simulink model "gm_sampleModel1890_2_sub"  (R2023a)
settings: Solver=VariableStepAuto  StartTime=0.0  StopTime=10.0  RelTol=1e-3
settings Model: Creator=user1  LastModifiedBy=user1
settings OptimizationCC: BlockReduction=off  ConditionallyExecuteInputs=off
settings DebuggingCC: InheritedTsInSrcMsg=none

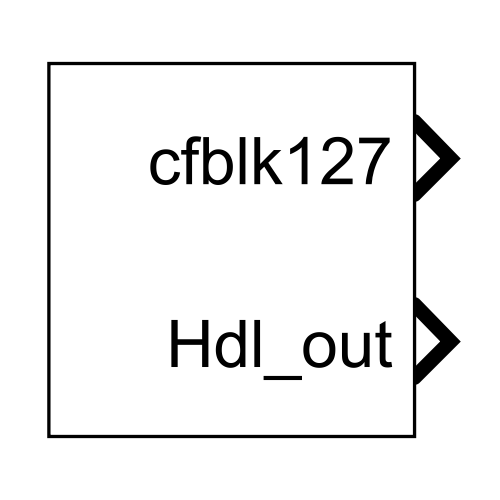
[thumbnail: Simulink's stored preview of the top-level diagram]
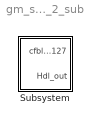
== system gm_sampleModel1890_2_sub ==
  Subsystem : Subsystem

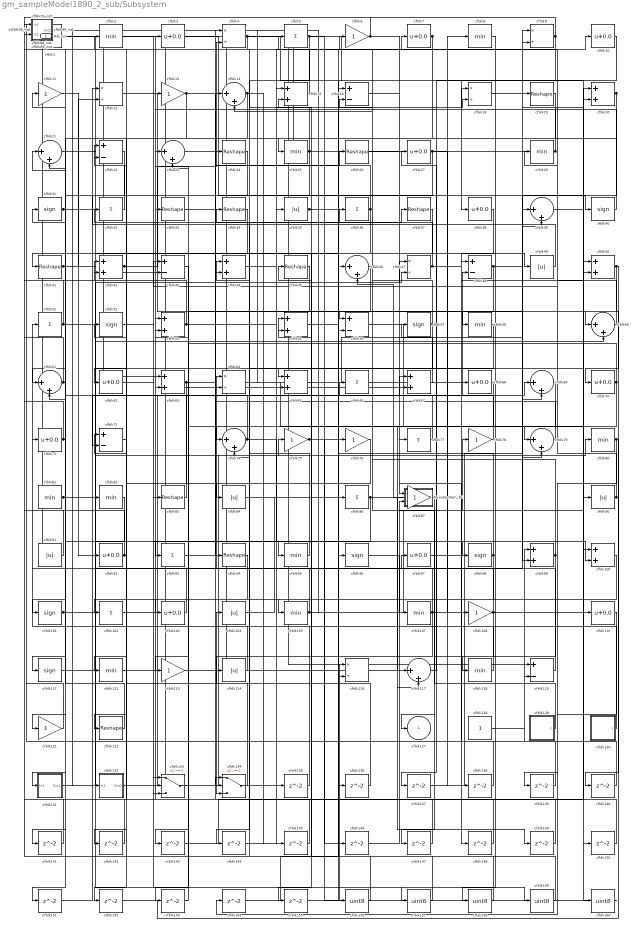
== system gm_sampleModel1890_2_sub/Subsystem ==
  Mysubsystem_36 : Subsystem
  cfblk{1,5,32,36,51,66,77,86,93,102} (10 alike) : Sum  Inputs=+  OutDataTypeStr=uint8
  cfblk{3,7,10,27,38,62,68,70..71,92,97,103,110} (13 alike) : Bias  Bias=0.0  SaturateOnIntegerOverflow=off
  cfblk{15,20,42,44,50,53,55,63,65,67,99..100} (12 alike) : Sum  OutDataTypeStr=uint8
  cfblk{31,40,52,57,96,98,101,111} (8 alike) : Signum
  cfblk{35,49,84,90..91,104,114} (7 alike) : Abs  OutDataTypeStr=uint8  SaturateOnIntegerOverflow=off
  cfblk{2,8,25,29,58,80..82,95,105,107,112,118} (13 alike) : MinMax  OutDataTypeStr=uint8
  cfblk{6,11,13,75..76,78,87,108,113,121} (10 alike) : Gain  OutDataTypeStr=uint8
  cfblk109_inst : Subsystem
  cfblk115_inst : Subsystem
  cfblk{4,9,12,18,47,64,116} (7 alike) : Product  Inputs=*/  OutDataTypeStr=uint8  RndMeth=Zero  SaturateOnIntegerOverflow=on
  cfblk{14,21,23,39,46,60..61,69,74,79,117} (11 alike) : Sum  Inputs=|++  OutDataTypeStr=uint8
  cfblk{16,22,43,48,56,72,119} (7 alike) : Sum  Inputs=+-  OutDataTypeStr=uint8
  cfblk120_inst : Subsystem
  cfblk{19,24,26,33..34,37,41,45,83,94,122} (11 alike) : Reshape
  cfblk128 : Constant  OutDataTypeStr=uint8  SampleTime=-1
  cfblk129 : Subsystem  mask(Counter Free-Running){NumBits=double(16), tsamp=double(-1)}
      mask prompts: NumBits "Simulink:masks:NumberOfBits_MP"; tsamp "Simulink:masks:SampleTime_MP"
      mask help: Simulink:masks:CounterFreeRunning_MD
  cfblk130 : Subsystem  mask(Counter Free-Running){NumBits=double(16), tsamp=double(-1)}
      mask prompts: NumBits "Simulink:masks:NumberOfBits_MP"; tsamp "Simulink:masks:SampleTime_MP"
      mask help: Simulink:masks:CounterFreeRunning_MD
  cfblk131 : Subsystem
  cfblk132 : Subsystem
  cfblk133 : Switch  OutDataTypeStr=uint8  SaturateOnIntegerOverflow=off  InputSameDT=off
  cfblk134 : Switch  OutDataTypeStr=uint8  SaturateOnIntegerOverflow=off  InputSameDT=off
  cfblk{135..155} (21 alike) : Delay  SampleTime=1
  cfblk{156..160} (5 alike) : DataTypeConversion  OutDataTypeStr=uint8  SaturateOnIntegerOverflow=off  RndMeth=Floor
  cfblk17_inst : Subsystem
  cfblk30_inst : Subsystem
  cfblk59_inst : Subsystem
  cfblk73_inst : Subsystem
  cfblk85_inst : Subsystem
  cfblk88_inst : Subsystem
  cfblk89_inst : Subsystem
  cfblk127 : Outport  OutDataTypeStr=uint8  SampleTime=1  VectorParamsAs1DForOutWhenUnconnected=off
  Hdl_out : Outport  Port=2  OutDataTypeStr=uint8  SampleTime=1
  wires:
  Mysubsystem_36/1(cfblk127) -> cfblk127/1
  cfblk1/1 -> cfblk159/1
  cfblk10/1 -> cfblk137/1
  cfblk100/1 -> cfblk105/1
  cfblk101/1 -> cfblk60/2, cfblk75/1, cfblk47/2
  cfblk102/1 -> cfblk3/1
  cfblk103/1 -> cfblk53/1
  cfblk104/1 -> cfblk86/1
  cfblk105/1 -> cfblk78/1, cfblk51/1
  cfblk107/1 -> cfblk15/2, cfblk134/3, cfblk8/1
  cfblk108/1 -> cfblk64/1, cfblk147/1
  cfblk109_inst/1(out1) -> cfblk63/1
  cfblk11/1 -> cfblk92/1
  cfblk110/1 -> cfblk154/1
  cfblk111/1 -> Mysubsystem_36/2(In2)
  cfblk112/1 -> cfblk97/1
  cfblk113/1 -> cfblk80/1
  cfblk114/1 -> cfblk71/1
  cfblk115_inst/1(out1) -> cfblk117/1
  cfblk116/1 -> cfblk87/1
  cfblk117/1 -> cfblk27/1
  cfblk118/1 -> cfblk61/2
  cfblk119/1 -> cfblk45/1
  cfblk12/1 -> cfblk56/1
  cfblk120_inst/1(out1) -> cfblk135/1
  cfblk121/1 -> cfblk85_inst/1(in1)
  cfblk122/1 -> cfblk11/1
  cfblk128/1 -> cfblk99/1
  cfblk129/1(y) -> cfblk36/1
  cfblk13/1 -> cfblk94/1, cfblk152/1
  cfblk130/1(y) -> cfblk44/1
  cfblk131/1(Out1) -> cfblk35/1
  cfblk132/1(Out1) -> cfblk48/2
  cfblk133/1 -> cfblk39/1
  cfblk134/1 -> cfblk104/1
  cfblk135/1 -> cfblk42/1
  cfblk136/1 -> cfblk72/1
  cfblk137/1 -> cfblk9/2
  cfblk138/1 -> cfblk115_inst/2(in2)
  cfblk139/1 -> cfblk48/1
  cfblk14/1 -> cfblk21/2, cfblk145/1
  cfblk140/1 -> cfblk119/2
  cfblk141/1 -> cfblk109_inst/1(in1)
  cfblk142/1 -> cfblk59_inst/1(in1)
  cfblk143/1 -> cfblk20/2
  cfblk144/1 -> cfblk18/2
  cfblk145/1 -> cfblk22/1
  cfblk146/1 -> cfblk50/2
  cfblk147/1 -> cfblk63/2
  cfblk148/1 -> cfblk134/1
  cfblk149/1 -> cfblk89_inst/2(in2)
  cfblk15/1 -> cfblk73_inst/1(in1)
  cfblk150/1 -> cfblk23/1
  cfblk151/1 -> cfblk69/1
  cfblk152/1 -> cfblk60/1
  cfblk153/1 -> cfblk53/2
  cfblk154/1 -> cfblk46/1
  cfblk155/1 -> cfblk116/1
  cfblk156/1 -> cfblk34/1
  cfblk157/1 -> cfblk55/1
  cfblk158/1 -> cfblk55/2
  cfblk159/1 -> cfblk109_inst/2(in2)
  cfblk16/1 -> cfblk77/1
  cfblk160/1 -> cfblk1/1
  cfblk17_inst/1(out1) -> cfblk30_inst/2(in2)
  cfblk18/1 -> cfblk19/1
  cfblk19/1 -> cfblk62/1
  cfblk2/1 -> cfblk133/1
  cfblk20/1 -> cfblk99/2, cfblk25/1
  cfblk21/1 -> cfblk136/1
  cfblk22/1 -> cfblk72/2
  cfblk23/1 -> cfblk44/2
  cfblk24/1 -> cfblk131/1(In1)
  cfblk25/1 -> cfblk30_inst/1(in1), cfblk122/1
  cfblk26/1 -> cfblk40/1
  cfblk27/1 -> cfblk84/1, cfblk138/1
  cfblk29/1 -> cfblk13/1, Hdl_out/1
  cfblk3/1 -> cfblk69/2
  cfblk30_inst/1(out1) -> cfblk91/1
  cfblk31/1 -> cfblk76/1, cfblk121/1
  cfblk32/1 -> cfblk22/2
  cfblk33/1 -> cfblk26/1
  cfblk34/1 -> cfblk141/1
  cfblk35/1 -> cfblk79/1, cfblk100/2
  cfblk36/1 -> cfblk41/1, cfblk16/2, cfblk4/2
  cfblk37/1 -> cfblk65/1
  cfblk38/1 -> cfblk61/1
  cfblk39/1 -> cfblk90/1
  cfblk4/1 -> cfblk96/1, cfblk85_inst/2(in2), cfblk150/1
  cfblk40/1 -> cfblk14/1
  cfblk41/1 -> cfblk160/1, cfblk12/2
  cfblk42/1 -> cfblk79/2, cfblk24/1
  cfblk43/1 -> cfblk143/1
  cfblk44/1 -> cfblk7/1
  cfblk45/1 -> cfblk103/1
  cfblk46/1 -> cfblk95/1
  cfblk47/1 -> cfblk49/1, cfblk4/1, cfblk2/1
  cfblk48/1 -> cfblk56/2, cfblk20/1
  cfblk49/1 -> cfblk12/1
  cfblk5/1 -> cfblk38/1, cfblk144/1
  cfblk50/1 -> cfblk70/1, cfblk93/1
  cfblk51/1 -> cfblk73_inst/2(in2), cfblk114/1
  cfblk52/1 -> cfblk157/1
  cfblk53/1 -> cfblk120_inst/1(in1), cfblk18/1
  cfblk55/1 -> cfblk156/1
  cfblk56/1 -> cfblk100/1
  cfblk57/1 -> cfblk74/2, cfblk17_inst/2(in2), cfblk14/2
  cfblk58/1 -> cfblk155/1
  cfblk59_inst/1(out1) -> cfblk110/1, cfblk132/1(In1)
  cfblk6/1 -> cfblk17_inst/1(in1), cfblk148/1
  cfblk60/1 -> cfblk29/1
  cfblk61/1 -> cfblk21/1, cfblk120_inst/2(in2)
  cfblk62/1 -> cfblk83/1
  cfblk63/1 -> cfblk47/1, cfblk102/1
  cfblk64/1 -> cfblk117/2
  cfblk65/1 -> cfblk39/2
  cfblk66/1 -> Mysubsystem_36/1(In1)
  cfblk67/1 -> cfblk57/1
  cfblk68/1 -> cfblk74/1
  cfblk69/1 -> cfblk116/2
  cfblk7/1 -> cfblk134/2, cfblk101/1
  cfblk70/1 -> cfblk23/2, cfblk113/1
  cfblk71/1 -> cfblk88_inst/2(in2), cfblk151/1
  cfblk72/1 -> cfblk42/2
  cfblk73_inst/1(out1) -> cfblk67/2, cfblk65/2
  cfblk74/1 -> cfblk98/1, cfblk33/1
  cfblk75/1 -> cfblk67/1, cfblk146/1
  cfblk76/1 -> cfblk112/1
  cfblk77/1 -> cfblk52/1
  cfblk78/1 -> cfblk15/1
  cfblk79/1 -> cfblk9/1
  cfblk8/1 -> cfblk158/1
  cfblk80/1 -> cfblk140/1, cfblk139/1
  cfblk81/1 -> cfblk108/1, cfblk82/1
  cfblk82/1 -> cfblk111/1
  cfblk83/1 -> cfblk59_inst/2(in2)
  cfblk84/1 -> cfblk10/1
  cfblk85_inst/1(out1) -> cfblk43/2, cfblk81/1
  cfblk86/1 -> cfblk133/2, cfblk6/1, cfblk149/1
  cfblk87/1 -> cfblk46/2
  cfblk88_inst/1(out1) -> cfblk68/1
  cfblk89_inst/1(out1) -> cfblk119/1
  cfblk9/1 -> cfblk89_inst/1(in1), cfblk58/1
  cfblk90/1 -> cfblk43/1, cfblk64/2, cfblk5/1
  cfblk91/1 -> cfblk115_inst/1(in1)
  cfblk92/1 -> cfblk88_inst/1(in1), cfblk31/1
  cfblk93/1 -> cfblk37/1
  cfblk94/1 -> cfblk153/1
  cfblk95/1 -> cfblk32/1
  cfblk96/1 -> cfblk107/1
  cfblk97/1 -> cfblk50/1
  cfblk98/1 -> cfblk16/1, cfblk133/3, cfblk142/1
  cfblk99/1 -> cfblk118/1, cfblk66/1

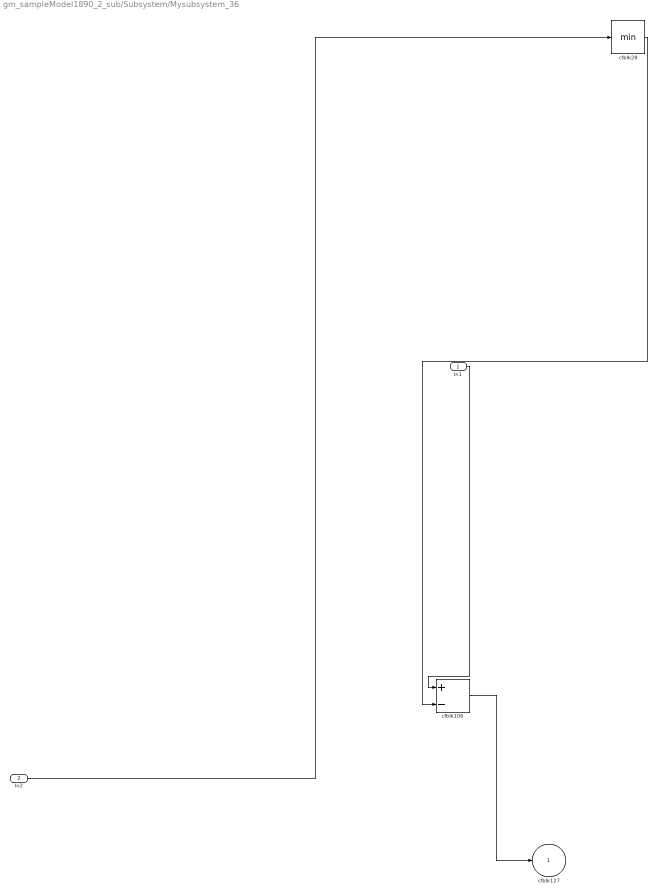
== system gm_sampleModel1890_2_sub/Subsystem/Mysubsystem_36 ==
  In1 : Inport  OutDataTypeStr=uint8  PortDimensions=1  SampleTime=1
  In2 : Inport  Port=2  OutDataTypeStr=uint8  PortDimensions=1  SampleTime=1
  cfblk106 : Sum  Inputs=+-
  cfblk28 : MinMax
  cfblk127 : Outport  SampleTime=1  VectorParamsAs1DForOutWhenUnconnected=off
  wires:
  In1/1 -> cfblk106/1
  In2/1 -> cfblk28/1
  cfblk106/1 -> cfblk127/1
  cfblk28/1 -> cfblk106/2

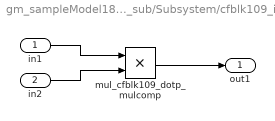
== system gm_sampleModel1890_2_sub/Subsystem/cfblk109_inst ==
  in1 : Inport  OutDataTypeStr=uint8  SampleTime=1
  in2 : Inport  Port=2  OutDataTypeStr=uint8  SampleTime=1
  mul_cfblk109_dotp_mulcomp : Product  Inputs=**  OutDataTypeStr=uint8  SampleTime=1
  out1 : Outport  OutDataTypeStr=uint8  SampleTime=1
  wires:
  in1/1 -> mul_cfblk109_dotp_mulcomp/1
  in2/1 -> mul_cfblk109_dotp_mulcomp/2
  mul_cfblk109_dotp_mulcomp/1 -> out1/1

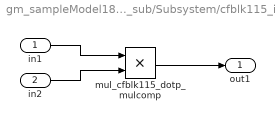
== system gm_sampleModel1890_2_sub/Subsystem/cfblk115_inst ==
  in1 : Inport  OutDataTypeStr=uint8  SampleTime=1
  in2 : Inport  Port=2  OutDataTypeStr=uint8  SampleTime=1
  mul_cfblk115_dotp_mulcomp : Product  Inputs=**  OutDataTypeStr=uint8  SampleTime=1
  out1 : Outport  OutDataTypeStr=uint8  SampleTime=1
  wires:
  in1/1 -> mul_cfblk115_dotp_mulcomp/1
  in2/1 -> mul_cfblk115_dotp_mulcomp/2
  mul_cfblk115_dotp_mulcomp/1 -> out1/1

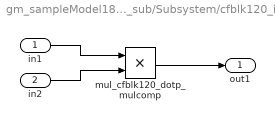
== system gm_sampleModel1890_2_sub/Subsystem/cfblk120_inst ==
  in1 : Inport  OutDataTypeStr=uint8  SampleTime=1
  in2 : Inport  Port=2  OutDataTypeStr=uint8  SampleTime=1
  mul_cfblk120_dotp_mulcomp : Product  Inputs=**  OutDataTypeStr=uint8  SampleTime=1
  out1 : Outport  OutDataTypeStr=uint8  SampleTime=1
  wires:
  in1/1 -> mul_cfblk120_dotp_mulcomp/1
  in2/1 -> mul_cfblk120_dotp_mulcomp/2
  mul_cfblk120_dotp_mulcomp/1 -> out1/1

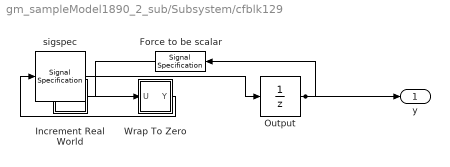
== system gm_sampleModel1890_2_sub/Subsystem/cfblk129 ==
  Force to be scalar : SignalSpecification  DisableCoverage=on  Dimensions=1
  Increment Real World : Subsystem  mask(Real World Value Increment){}
      mask help: Simulink:masks:RealWorldValueIncrement_MD
      mask Display: disp('V++')
  Output : UnitDelay  InitialCondition=0.0  SampleTime=tsamp  HasFrameUpgradeWarning=on
  Wrap To Zero : Subsystem  mask(Wrap To Zero){Threshold=double(65535)}
      mask prompts: Threshold "Simulink:masks:Threshold_MP"
      mask help: Simulink:masks:WrapToZero_MD
  sigspec : SignalSpecification  OutDataTypeStr=uint16  Dimensions=1
  y : Outport  SampleTime=1
  wires:
  Force to be scalar/1 -> Increment Real World/1(u)
  Increment Real World/1(y) -> Wrap To Zero/1(U)
  Output/1 -> Force to be scalar/1, y/1
  Wrap To Zero/1(Y) -> sigspec/1
  sigspec/1 -> Output/1

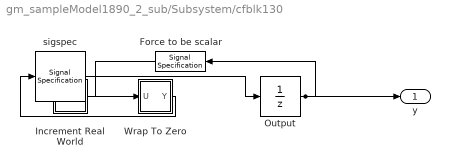
== system gm_sampleModel1890_2_sub/Subsystem/cfblk130 ==
  Force to be scalar : SignalSpecification  DisableCoverage=on  Dimensions=1
  Increment Real World : Subsystem  mask(Real World Value Increment){}
      mask help: Simulink:masks:RealWorldValueIncrement_MD
      mask Display: disp('V++')
  Output : UnitDelay  InitialCondition=0.0  SampleTime=tsamp  HasFrameUpgradeWarning=on
  Wrap To Zero : Subsystem  mask(Wrap To Zero){Threshold=double(65535)}
      mask prompts: Threshold "Simulink:masks:Threshold_MP"
      mask help: Simulink:masks:WrapToZero_MD
  sigspec : SignalSpecification  OutDataTypeStr=uint16  Dimensions=1
  y : Outport  SampleTime=1
  wires:
  Force to be scalar/1 -> Increment Real World/1(u)
  Increment Real World/1(y) -> Wrap To Zero/1(U)
  Output/1 -> Force to be scalar/1, y/1
  Wrap To Zero/1(Y) -> sigspec/1
  sigspec/1 -> Output/1

== system gm_sampleModel1890_2_sub/Subsystem/cfblk131 ==
  In1 : Inport  OutDataTypeStr=uint8  PortDimensions=1  SampleTime=1
  Out1 : Outport  SampleTime=1
  wires:
  In1/1 -> Out1/1

== system gm_sampleModel1890_2_sub/Subsystem/cfblk132 ==
  In1 : Inport  OutDataTypeStr=uint8  PortDimensions=1  SampleTime=1
  Out1 : Outport  SampleTime=1
  wires:
  In1/1 -> Out1/1

== system gm_sampleModel1890_2_sub/Subsystem/cfblk17_inst ==
  in1 : Inport  OutDataTypeStr=uint8  SampleTime=1
  in2 : Inport  Port=2  OutDataTypeStr=uint8  SampleTime=1
  mul_cfblk17_dotp_mulcomp : Product  Inputs=**  OutDataTypeStr=uint8  SampleTime=1
  out1 : Outport  OutDataTypeStr=uint8  SampleTime=1
  wires:
  in1/1 -> mul_cfblk17_dotp_mulcomp/1
  in2/1 -> mul_cfblk17_dotp_mulcomp/2
  mul_cfblk17_dotp_mulcomp/1 -> out1/1

== system gm_sampleModel1890_2_sub/Subsystem/cfblk30_inst ==
  in1 : Inport  OutDataTypeStr=uint8  SampleTime=1
  in2 : Inport  Port=2  OutDataTypeStr=uint8  SampleTime=1
  mul_cfblk30_dotp_mulcomp : Product  Inputs=**  OutDataTypeStr=uint8  SampleTime=1
  out1 : Outport  OutDataTypeStr=uint8  SampleTime=1
  wires:
  in1/1 -> mul_cfblk30_dotp_mulcomp/1
  in2/1 -> mul_cfblk30_dotp_mulcomp/2
  mul_cfblk30_dotp_mulcomp/1 -> out1/1

== system gm_sampleModel1890_2_sub/Subsystem/cfblk59_inst ==
  in1 : Inport  OutDataTypeStr=uint8  SampleTime=1
  in2 : Inport  Port=2  OutDataTypeStr=uint8  SampleTime=1
  mul_cfblk59_dotp_mulcomp : Product  Inputs=**  OutDataTypeStr=uint8  SampleTime=1
  out1 : Outport  OutDataTypeStr=uint8  SampleTime=1
  wires:
  in1/1 -> mul_cfblk59_dotp_mulcomp/1
  in2/1 -> mul_cfblk59_dotp_mulcomp/2
  mul_cfblk59_dotp_mulcomp/1 -> out1/1

== system gm_sampleModel1890_2_sub/Subsystem/cfblk73_inst ==
  in1 : Inport  OutDataTypeStr=uint8  SampleTime=1
  in2 : Inport  Port=2  OutDataTypeStr=uint8  SampleTime=1
  mul_cfblk73_dotp_mulcomp : Product  Inputs=**  OutDataTypeStr=uint8  SampleTime=1
  out1 : Outport  OutDataTypeStr=uint8  SampleTime=1
  wires:
  in1/1 -> mul_cfblk73_dotp_mulcomp/1
  in2/1 -> mul_cfblk73_dotp_mulcomp/2
  mul_cfblk73_dotp_mulcomp/1 -> out1/1

== system gm_sampleModel1890_2_sub/Subsystem/cfblk85_inst ==
  in1 : Inport  OutDataTypeStr=uint8  SampleTime=1
  in2 : Inport  Port=2  OutDataTypeStr=uint8  SampleTime=1
  mul_cfblk85_dotp_mulcomp : Product  Inputs=**  OutDataTypeStr=uint8  SampleTime=1
  out1 : Outport  OutDataTypeStr=uint8  SampleTime=1
  wires:
  in1/1 -> mul_cfblk85_dotp_mulcomp/1
  in2/1 -> mul_cfblk85_dotp_mulcomp/2
  mul_cfblk85_dotp_mulcomp/1 -> out1/1

== system gm_sampleModel1890_2_sub/Subsystem/cfblk88_inst ==
  in1 : Inport  OutDataTypeStr=uint8  SampleTime=1
  in2 : Inport  Port=2  OutDataTypeStr=uint8  SampleTime=1
  mul_cfblk88_dotp_mulcomp : Product  Inputs=**  OutDataTypeStr=uint8  SampleTime=1
  out1 : Outport  OutDataTypeStr=uint8  SampleTime=1
  wires:
  in1/1 -> mul_cfblk88_dotp_mulcomp/1
  in2/1 -> mul_cfblk88_dotp_mulcomp/2
  mul_cfblk88_dotp_mulcomp/1 -> out1/1

== system gm_sampleModel1890_2_sub/Subsystem/cfblk89_inst ==
  in1 : Inport  OutDataTypeStr=uint8  SampleTime=1
  in2 : Inport  Port=2  OutDataTypeStr=uint8  SampleTime=1
  mul_cfblk89_dotp_mulcomp : Product  Inputs=**  OutDataTypeStr=uint8  SampleTime=1
  out1 : Outport  OutDataTypeStr=uint8  SampleTime=1
  wires:
  in1/1 -> mul_cfblk89_dotp_mulcomp/1
  in2/1 -> mul_cfblk89_dotp_mulcomp/2
  mul_cfblk89_dotp_mulcomp/1 -> out1/1

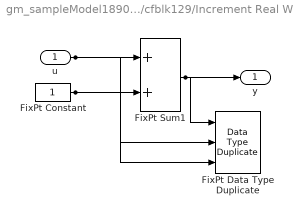
== system gm_sampleModel1890_2_sub/Subsystem/cfblk129/Increment Real World ==
  u : Inport  OutDataTypeStr=uint16  SampleTime=1
  FixPt Constant : Constant  DisableCoverage=on  OutDataTypeStr=Inherit: Inherit via back propagation  SampleTime=-1
  FixPt Data Type Duplicate : DataTypeDuplicate  DisableCoverage=on  NumInputPorts=3
  FixPt Sum1 : Sum  InputSameDT=on  OutDataTypeStr=Inherit: Inherit via back propagation  LockScale=on
  y : Outport  SampleTime=1
  wires:
  u/1 -> FixPt Sum1/1, FixPt Data Type Duplicate/2
  FixPt Constant/1 -> FixPt Sum1/2, FixPt Data Type Duplicate/3
  FixPt Sum1/1 -> FixPt Data Type Duplicate/1, y/1

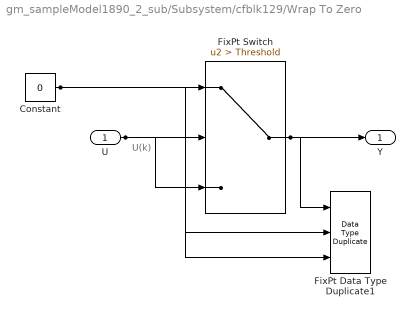
== system gm_sampleModel1890_2_sub/Subsystem/cfblk129/Wrap To Zero ==
  note: U(k)
  U : Inport  OutDataTypeStr=uint16  SampleTime=1
  Constant : Constant  DisableCoverage=on  Value=0  OutDataTypeStr=Inherit: Inherit via back propagation  SampleTime=-1
  FixPt Data Type Duplicate1 : DataTypeDuplicate  DisableCoverage=on  NumInputPorts=3
  FixPt Switch : Switch  Criteria=u2 > Threshold  Threshold=Threshold  OutDataTypeStr=Inherit: Inherit via back propagation  ZeroCross=off  SaturateOnIntegerOverflow=off  InputSameDT=off
  Y : Outport  SampleTime=1
  wires:
  U/1 -> FixPt Switch/3, FixPt Switch/2, FixPt Data Type Duplicate1/2
  Constant/1 -> FixPt Switch/1, FixPt Data Type Duplicate1/3
  FixPt Switch/1 -> FixPt Data Type Duplicate1/1, Y/1

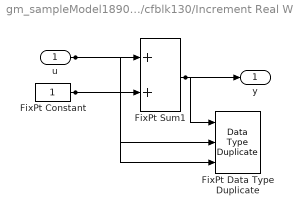
== system gm_sampleModel1890_2_sub/Subsystem/cfblk130/Increment Real World ==
  u : Inport  OutDataTypeStr=uint16  SampleTime=1
  FixPt Constant : Constant  DisableCoverage=on  OutDataTypeStr=Inherit: Inherit via back propagation  SampleTime=-1
  FixPt Data Type Duplicate : DataTypeDuplicate  DisableCoverage=on  NumInputPorts=3
  FixPt Sum1 : Sum  InputSameDT=on  OutDataTypeStr=Inherit: Inherit via back propagation  LockScale=on
  y : Outport  SampleTime=1
  wires:
  u/1 -> FixPt Sum1/1, FixPt Data Type Duplicate/2
  FixPt Constant/1 -> FixPt Sum1/2, FixPt Data Type Duplicate/3
  FixPt Sum1/1 -> FixPt Data Type Duplicate/1, y/1

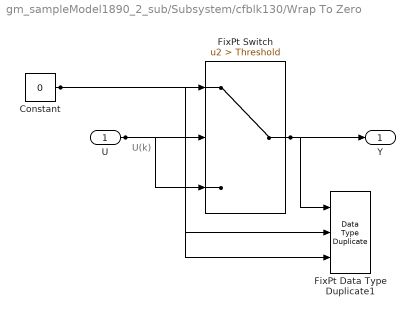
== system gm_sampleModel1890_2_sub/Subsystem/cfblk130/Wrap To Zero ==
  note: U(k)
  U : Inport  OutDataTypeStr=uint16  SampleTime=1
  Constant : Constant  DisableCoverage=on  Value=0  OutDataTypeStr=Inherit: Inherit via back propagation  SampleTime=-1
  FixPt Data Type Duplicate1 : DataTypeDuplicate  DisableCoverage=on  NumInputPorts=3
  FixPt Switch : Switch  Criteria=u2 > Threshold  Threshold=Threshold  OutDataTypeStr=Inherit: Inherit via back propagation  ZeroCross=off  SaturateOnIntegerOverflow=off  InputSameDT=off
  Y : Outport  SampleTime=1
  wires:
  U/1 -> FixPt Switch/3, FixPt Switch/2, FixPt Data Type Duplicate1/2
  Constant/1 -> FixPt Switch/1, FixPt Data Type Duplicate1/3
  FixPt Switch/1 -> FixPt Data Type Duplicate1/1, Y/1
